simulink model "modelo_no_linear_pid"  (R2022a)
settings: Solver=VariableStepAuto  StartTime=0.0  StopTime=100  RelTol=1e-3
values from neighbouring files (symbols this model uses):
  amplitude_entrada = 0.05    [ball_and_beam_pfc.m]
  bool_degrau = 1    [ball_and_beam_pfc.m]
  C = [0 0 1 0]    [ball_and_beam_pfc.m]
  C2_A = [X(7) X(5) X(3) X(1)]    [ball_and_beam_pfc.m]
  C2_M = [X(8) X(6) X(4) X(2)]    [ball_and_beam_pfc.m]
  g = 9.8    [ball_and_beam_pfc.m]    (also in nonlinear_ball_and_beam.m)
  Jv = (1/2) * mv * L^2    (= 0.058703125)    [ball_and_beam_pfc.m]    (also in nonlinear_ball_and_beam.m)
  L = 0.425    [ball_and_beam_pfc.m]    (also in nonlinear_ball_and_beam.m)
  Ls = f(8)/a(5)    [ball_and_beam_pfc.m]
  mb = 0.064    [ball_and_beam_pfc.m]    (also in nonlinear_ball_and_beam.m)
  mv = 0.65    [ball_and_beam_pfc.m]    (also in nonlinear_ball_and_beam.m)
libraries: vrlib x3
settings Model: Creator=Notebook_Artur  LastModifiedBy=Notebook_Artur

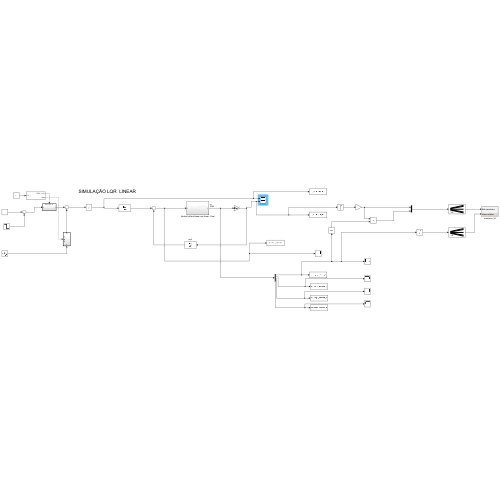
[thumbnail: Simulink's stored preview of the top-level diagram]
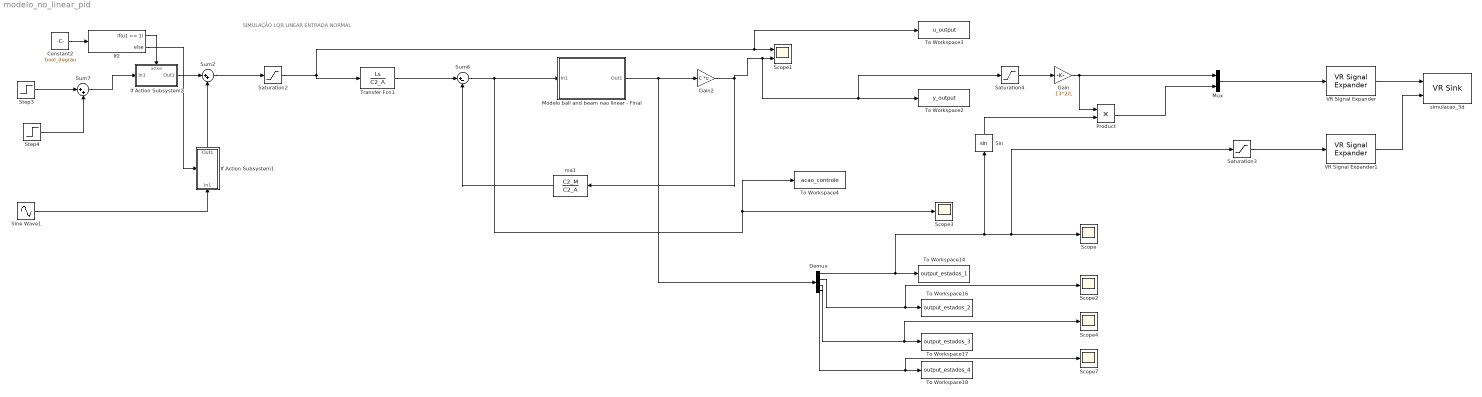
== system modelo_no_linear_pid ==
  note: SIMULAÇÃO LQR LINEAR ENTRADA NORMAL
  Constant2 : Constant  Value=bool_degrau
  Demux : Demux
  Gain : Gain  Gain=13*2/L
  Gain2 : Gain  Gain=C  Multiplication=Matrix(K*u)
  If Action Subsystem1 : Subsystem  TreatAsAtomicUnit=on
  If Action Subsystem2 : Subsystem  TreatAsAtomicUnit=on
  If2 : If  IfExpression=u1 == 1
  Modelo ball and beam nao linear - Final : Subsystem
  Mux : Mux  Inputs=2
  Product : Product
  Saturation2 : Saturate  UpperLimit=L/2  LowerLimit=-L/2
  Saturation3 : Saturate  UpperLimit=0.1  LowerLimit=-0.1
  Saturation4 : Saturate  UpperLimit=L/2  LowerLimit=0
  Scope{,2..4,7} (5 alike) : Scope
  Scope1 : Scope  NumInputPorts=2
  Sin : Trigonometry
  Sine Wave1 : Sin  Amplitude=amplitude_entrada  Frequency=0.1  SampleTime=0
  Step3 : Step  After=amplitude_entrada  SampleTime=0
  Step4 : Step  Time=100  After=-2*amplitude_entrada  SampleTime=0
  Sum2 : Sum  Inputs=|++
  Sum6 : Sum  Inputs=|+-
  Sum7 : Sum  Inputs=|++
  To Workspace14 : ToWorkspace  VariableName=output_estados_1  SaveFormat=Timeseries  SampleTime=-1
  To Workspace16 : ToWorkspace  VariableName=output_estados_2  SaveFormat=Timeseries  SampleTime=-1
  To Workspace17 : ToWorkspace  VariableName=output_estados_3  SaveFormat=Timeseries  SampleTime=-1
  To Workspace18 : ToWorkspace  VariableName=output_estados_4  SaveFormat=Timeseries  SampleTime=-1
  To Workspace2 : ToWorkspace  VariableName=y_output  SaveFormat=Timeseries  SampleTime=-1
  To Workspace3 : ToWorkspace  VariableName=u_output  SaveFormat=Timeseries  SampleTime=-1
  To Workspace4 : ToWorkspace  VariableName=acao_controle  SaveFormat=Timeseries  SampleTime=-1
  Transfer Fcn1 : TransferFcn  Numerator=Ls  Denominator=C2_A
  VR Signal Expander : vrlib/VR Signal Expander  outwidth=3  outidx=[1 3]
  VR Signal Expander1 : vrlib/VR Signal Expander  outwidth=4  outidx=[4]
  ma1 : TransferFcn  Numerator=C2_M  Denominator=C2_A
  simulacao_3d : vrlib/VR Sink  InstantiateOnLoad=on  SampleTime=0.1  ViewEnable=on  RemoteChange=off  RemoteView=off  FieldsWritten=Ball.translation.3.1.1.double#beam.rotation.4.1.1.double  WorldFileName=3d_ball_and_beam4.x3d  AutoView=on  VideoDimensions=[]  AllowVariableSize=off
  wires:
  Gain/1 -> Product/1, Mux/1
  Sum7/1 -> If Action Subsystem2/1(In1)
  Modelo ball and beam nao linear - Final/1(Out1) -> Demux/1, Gain2/1
  Mux/1 -> VR Signal Expander/1
  Sin/1 -> Product/2
  Step3/1 -> Sum7/1
  VR Signal Expander1/1 -> simulacao_3d/2
  Gain2/1 -> Saturation4/1, To Workspace2/1, Scope1/2, ma1/1
  Demux/1 -> Scope/1, Saturation3/1, Sin/1, To Workspace14/1
  Demux/2 -> Scope2/1, To Workspace16/1
  If2/1 -> If Action Subsystem2/Action
  Saturation3/1 -> VR Signal Expander1/1
  If Action Subsystem1/1(Out1) -> Sum2/2
  Product/1 -> Mux/2
  Constant2/1 -> If2/1
  Sum2/1 -> Saturation2/1
  Saturation2/1 -> To Workspace3/1, Scope1/1, Transfer Fcn1/1
  If2/2 -> If Action Subsystem1/Action
  Demux/3 -> Scope4/1, To Workspace17/1
  Sine Wave1/1 -> If Action Subsystem1/1(In1)
  If Action Subsystem2/1(Out1) -> Sum2/1
  Demux/4 -> Scope7/1, To Workspace18/1
  VR Signal Expander/1 -> simulacao_3d/1
  Saturation4/1 -> Gain/1
  Step4/1 -> Sum7/2
  Sum6/1 -> Modelo ball and beam nao linear - Final/1(In1), To Workspace4/1, Scope3/1
  Transfer Fcn1/1 -> Sum6/1
  ma1/1 -> Sum6/2

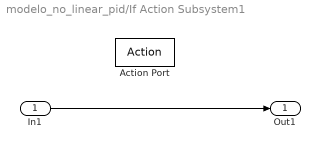
== system modelo_no_linear_pid/If Action Subsystem1 ==
  In1 : Inport
  Action Port : ActionPort  ActionPortLabel=else
  Out1 : Outport
  wires:
  In1/1 -> Out1/1

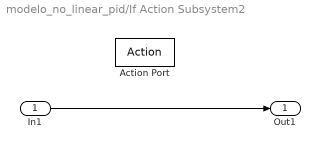
== system modelo_no_linear_pid/If Action Subsystem2 ==
  In1 : Inport
  Action Port : ActionPort  ActionPortLabel=if(u1 == 1)
  Out1 : Outport
  wires:
  In1/1 -> Out1/1

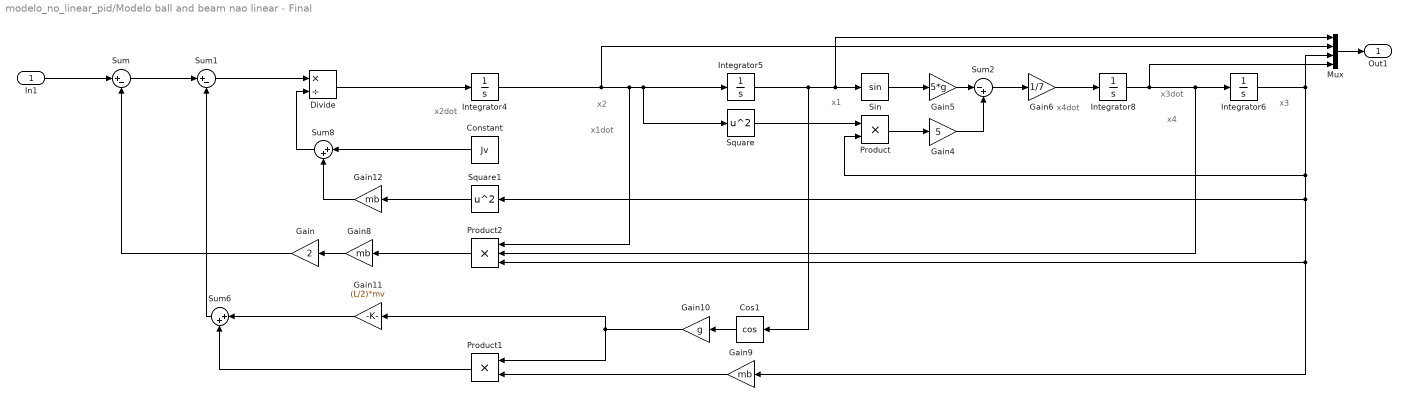
== system modelo_no_linear_pid/Modelo ball and beam nao linear - Final ==
  note: x3
  note: x3dot
  note: x4
  note: x4dot
  note: x1
  note: x1dot
  note: x2dot
  note: x2
  In1 : Inport
  Constant : Constant  Value=Jv
  Cos1 : Trigonometry  Operator=cos
  Divide : Product  Inputs=*/
  Gain : Gain  Gain=2
  Gain10 : Gain  Gain=g
  Gain11 : Gain  Gain=(L/2)*mv
  Gain12 : Gain  Gain=mb
  Gain4 : Gain  Gain=5
  Gain5 : Gain  Gain=5*g
  Gain6 : Gain  Gain=1/7
  Gain8 : Gain  Gain=mb
  Gain9 : Gain  Gain=mb
  Integrator{4..6,8} (4 alike) : Integrator
  Mux : Mux
  Product : Product
  Product1 : Product
  Product2 : Product  Inputs=3
  Sin : Trigonometry
  Square : Math  Operator=square
  Square1 : Math  Operator=square
  Sum : Sum  Inputs=|+-
  Sum1 : Sum  Inputs=|+-
  Sum2 : Sum  Inputs=|-+
  Sum6 : Sum  Inputs=|++
  Sum8 : Sum  Inputs=|++
  Out1 : Outport
  wires:
  Integrator8/1 -> Mux/4, Product2/2, Integrator6/1
  Integrator5/1 -> Sin/1, Mux/1, Cos1/1
  Sum6/1 -> Sum1/2
  Sum2/1 -> Gain6/1
  Gain10/1 -> Product1/1, Gain11/1
  Square/1 -> Product/1
  Integrator6/1 -> Mux/3, Gain9/1, Product2/3, Square1/1, Product/2
  Gain11/1 -> Sum6/1
  Gain12/1 -> Sum8/2
  Gain6/1 -> Integrator8/1
  Gain4/1 -> Sum2/2
  Gain9/1 -> Product1/2
  Cos1/1 -> Gain10/1
  Divide/1 -> Integrator4/1
  Product2/1 -> Gain8/1
  Product/1 -> Gain4/1
  Square1/1 -> Gain12/1
  Sum8/1 -> Divide/2
  Product1/1 -> Sum6/2
  Constant/1 -> Sum8/1
  Mux/1 -> Out1/1
  Gain5/1 -> Sum2/1
  Sin/1 -> Gain5/1
  Gain8/1 -> Gain/1
  Sum1/1 -> Divide/1
  Sum/1 -> Sum1/1
  Integrator4/1 -> Mux/2, Product2/1, Square/1, Integrator5/1
  In1/1 -> Sum/1
  Gain/1 -> Sum/2
